simulink model "ATWS"  (R2019b)
settings: Solver=FixedStepDiscrete  StartTime=0.0  StopTime=20  FixedStep=0.01  RelTol=1e-3
model workspace (MAT data in the model file):
  M_TIME_400MS = Simulink.Parameter
  M_TIME_400MS.Value = 40
  M_TIME_400MS.DataType = 'uint16'
  M_TIME_400MS.DocUnits = 'ms'
  M_TIME_400MS.Dimensions = [1 1]
  M_TIME_5S = Simulink.Parameter
  M_TIME_5S.Value = 500
  M_TIME_5S.DataType = 'uint16'
  M_TIME_5S.DocUnits = 's'
  M_TIME_5S.Dimensions = [1 1]
undefined symbols (not defined in the file): M_TIME_800MS
settings Model: Creator=seanryu  LastModifiedBy=bhisma
settings DataIOCC: ExternalInput=[t, CentralUnlockSw]  ReturnWorkspaceOutputs=off
settings OptimizationCC: DefaultParameterBehavior=Inlined  EfficientTunableParamExpr=on
settings DebuggingCC: ParameterTunabilityLossMsg=error  ArithmeticOperatorsInVariantConditions=warning
settings SFSimCC: SimUseLocalCustomCode=off  MATLABDynamicMemAlloc=off  CustomCodeUndefinedFunction=UseInterfaceOnly
settings RTWCC: SystemTargetFile=ert.tlc  GenCodeOnly=on  TemplateMakefile=ert_default_tmf  GenerateReport=on  RTWUseLocalCustomCode=off  IncludeHyperlinkInReport=on  LaunchReport=on  GenerateTraceInfo=on  GenerateTraceReport=on  GenerateTraceReportSl=on  GenerateTraceReportSf=on  GenerateTraceReportEml=on  GenerateCodeMetricsReport=on
settings CodeAppCC: ForceParamTrailComments=on  IgnoreCustomStorageClasses=off  OperatorAnnotations=on  SimulinkDataObjDesc=on  SFDataObjDesc=on  MATLABFcnDesc=on  InsertBlockDesc=on  StateflowObjectComments=on  MATLABSourceComments=on
settings ERTTargetCC: TargetLangStandard=C99 (ISO)  MultiwordLength=2048  GenerateSampleERTMain=on  SupportNonFinite=off  InlinedParameterPlacement=NonHierarchical  ERTCustomFileTemplate=example_file_process.tlc  IndentStyle=Allman  IndentSize=4

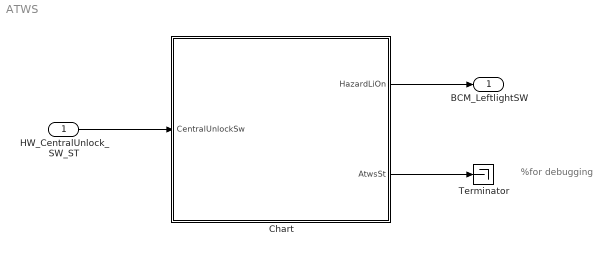
== system ATWS ==
  note: %for debugging
  HW_CentralUnlock_SW_ST : Inport
  Chart : Stateflow chart  TreatAsAtomicUnit=on
  Terminator : Terminator
  BCM_LeftlightSW : Outport
  wires:
  HW_CentralUnlock_SW_ST/1 -> Chart/1(CentralUnlockSw)
  Chart/1(HazardLiOn) -> BCM_LeftlightSW/1
  Chart/2(AtwsSt) -> Terminator/1

== stateflow chart ATWS/Chart ==
  settings: stateMachineType=MOORE_MACHINE
  note: %Ready
  state AtwsInit
    AtwsCnt = 1;
    %AtwsSt = 0;
    BlkngCnt = 0;
    BcmLeLiSt = 0;
    CycCnt = 0;
    LeLiCyc = 0;
  state AtwsCntr
    AtwsCnt = AtwsCnt + 1
  state AtwsEnaSt
    AtwsCnt = 0;
    AtwsSt = 1
    LeLiCyc = 1;
    HazardLiOn = 1;
  state AtwsDisSt
    AtwsCnt = 0;
    AtwsSt = 0
    LeLiCyc = 2;
    HazardLiOn = 1;
  state AtwsLiCntrl
    state LiOn
      BlkngCnt = BlkngCnt+1;
      HazardLiOn = 1;
    state LiOff
      BlkngCnt = BlkngCnt+1;
      HazardLiOn = 0;
    state LiCntrInit
      BlkngCnt = 0;
    state LiCycCntr
      CycCnt = CycCnt + 1;
    state LiTerm
      BcmLeLiSt = 1;
      CycCnt = 0;
    (default) -> LiOn
    (junction 278) -> LiOn
    LiCntrInit -> (junction 278)
    LiOn -> LiOff : [BlkngCnt >= (M_TIME_400MS-1)]
    LiOff -> LiCycCntr : [BlkngCnt >= (M_TIME_800MS-1)]
    (junction 280) -> LiCntrInit
    LiCycCntr -> (junction 272)
    (junction 272) -> (junction 280) [order 1] : [(AtwsSt == 0) && (CycCnt < LeLiCyc)]
    (junction 272) -> LiTerm [order 2]
    LiTerm -> (junction 267)
  (default) -> AtwsInit
  AtwsCntr -> AtwsEnaSt [order 2] : [(AtwsCnt >= M_TIME_5S) && (AtwsSt == 0)]
  AtwsInit -> AtwsCntr : [CentralUnlockSw == 1]
  AtwsCntr -> AtwsInit [order 1] : [CentralUnlockSw == 0]
  (junction 238) -> AtwsInit
  AtwsCntr -> AtwsDisSt [order 3] : [(AtwsCnt >= M_TIME_5S) && (AtwsSt == 1)]
  AtwsEnaSt -> AtwsLiCntrl
  AtwsDisSt -> AtwsLiCntrl
  AtwsLiCntrl -> (junction 240)
  (junction 240) -> (junction 238) : [BcmLeLiSt == 1]
  data: AtwsCnt local =0; HazardLiOn output; BcmLeLiSt local; M_TIME_5S parameter double; M_TIME_800MS parameter; M_TIME_400MS parameter; LightSt local; CentralUnlockSw input; BlkngCnt local; LeLiCyc local; CycCnt local =0; AtwsSt output =0
